simulink model "helicopter"  (R2023b)
settings: Solver=VariableStepAuto  StartTime=0.0  StopTime=20  MaxStep=0.01  RelTol=1e-5
undefined symbols (not defined in the file): A, A_obs, B, B_alt, B_obs, C, C_obs, E_alt, K_act_b, K_act_f, K_f_lqr, K_lqr, L, M_inv_alt, sim_nonlinear, u0, x0
libraries: cstblocks x2, simulink x2
settings Model: Creator=torb  LastModifiedBy=torb

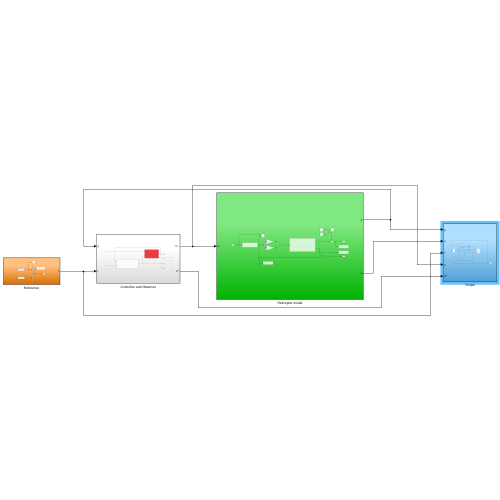
[thumbnail: Simulink's stored preview of the top-level diagram]
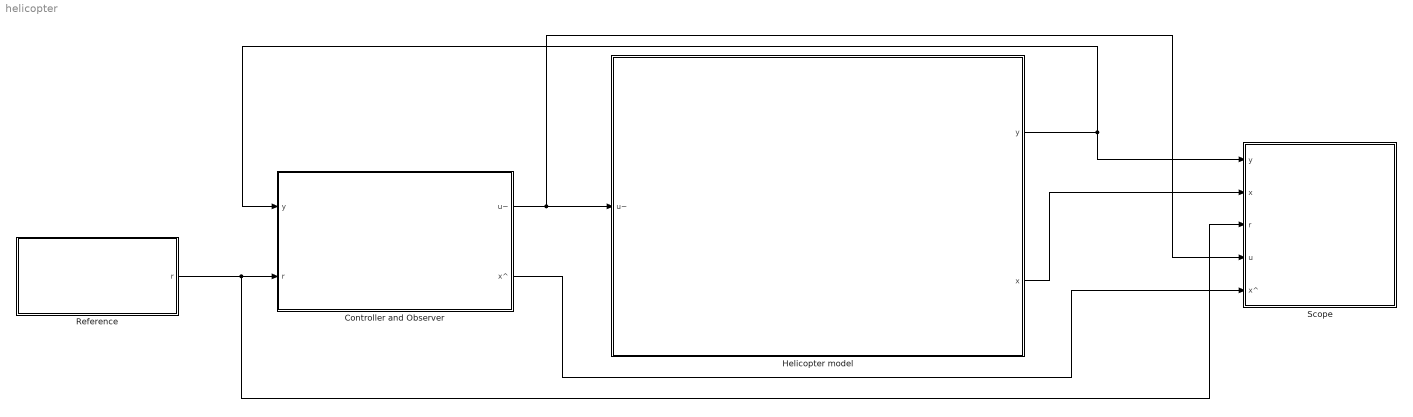
== system helicopter ==
  Controller and Observer : Subsystem
  Helicopter model : Subsystem
  Reference : Subsystem
  Scope : Subsystem
  wires:
  Helicopter model/1(y) -> Scope/1(y), Controller and Observer/1(y)
  Reference/1(r) -> Scope/3(r), Controller and Observer/2(r)
  Helicopter model/2(x) -> Scope/2(x)
  Controller and Observer/1(u~) -> Scope/4(u), Helicopter model/1(u~)
  Controller and Observer/2(x^) -> Scope/5(x^)

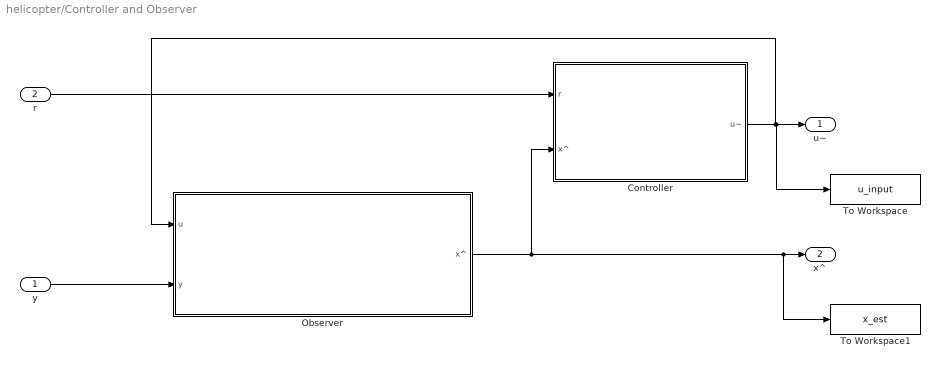
== system helicopter/Controller and Observer ==
  y : Inport
  r : Inport  Port=2
  Controller : Subsystem
  Observer : Subsystem
  To Workspace : ToWorkspace  VariableName=u_input  SaveFormat=Timeseries  SampleTime=-1
  To Workspace1 : ToWorkspace  VariableName=x_est  SaveFormat=Timeseries  SampleTime=-1
  u~ : Outport
  x^ : Outport  Port=2
  wires:
  Controller/1(u~) -> To Workspace/1, u~/1, Observer/1(u)
  Observer/1(x^) -> x^/1, To Workspace1/1, Controller/2(x^)
  r/1 -> Controller/1(r)
  y/1 -> Observer/2(y)

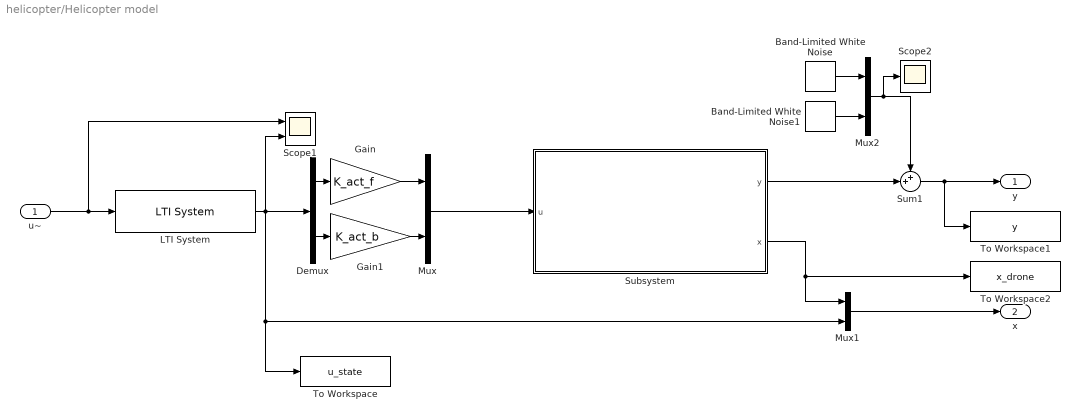
== system helicopter/Helicopter model ==
  u~ : Inport
  Band-Limited White Noise : simulink/Sources/Band-Limited White Noise  Cov=noise_power  Ts=0.01  seed=[23341]
  Band-Limited White Noise1 : simulink/Sources/Band-Limited White Noise  Cov=noise_power  Ts=0.01  seed=[231]
  Demux : Demux  Outputs=2
  Gain : Gain  Gain=K_act_f
  Gain1 : Gain  Gain=K_act_b
  LTI System : cstblocks/LTI System  sys=G_act_real  IC=[]  PadeOrder=0
  Mux : Mux  Inputs=2
  Mux1 : Mux  Inputs=2
  Mux2 : Mux  Inputs=2
  Scope1 : Scope  NumInputPorts=2
  Scope2 : Scope
  Subsystem : Subsystem
  Sum1 : Sum  Inputs=++|
  To Workspace : ToWorkspace  VariableName=u_state  SaveFormat=Timeseries  SampleTime=-1
  To Workspace1 : ToWorkspace  VariableName=y  SaveFormat=Timeseries  SampleTime=-1
  To Workspace2 : ToWorkspace  VariableName=x_drone  SaveFormat=Timeseries  SampleTime=-1
  y : Outport
  x : Outport  Port=2
  wires:
  u~/1 -> LTI System/1, Scope1/1
  LTI System/1 -> Demux/1, Mux1/2, To Workspace/1, Scope1/2
  Demux/2 -> Gain1/1
  Demux/1 -> Gain/1
  Gain/1 -> Mux/1
  Gain1/1 -> Mux/2
  Mux1/1 -> x/1
  Band-Limited White Noise/1 -> Mux2/1
  Band-Limited White Noise1/1 -> Mux2/2
  Mux2/1 -> Sum1/1, Scope2/1
  Sum1/1 -> y/1, To Workspace1/1
  Subsystem/2(x) -> Mux1/1, To Workspace2/1
  Mux/1 -> Subsystem/1(u)
  Subsystem/1(y) -> Sum1/2

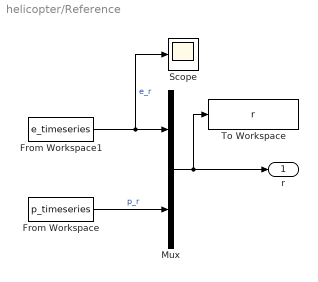
== system helicopter/Reference ==
  From Workspace : FromWorkspace  VariableName=p_timeseries
  From Workspace1 : FromWorkspace  VariableName=e_timeseries
  Mux : Mux  Inputs=2
  Scope : Scope
  To Workspace : ToWorkspace  VariableName=r  SaveFormat=Timeseries  SampleTime=-1
  r : Outport
  wires:
  Mux/1 -> To Workspace/1, r/1
  From Workspace/1 -> Mux/2  "p_r"
  From Workspace1/1 -> Mux/1, Scope/1  "e_r"

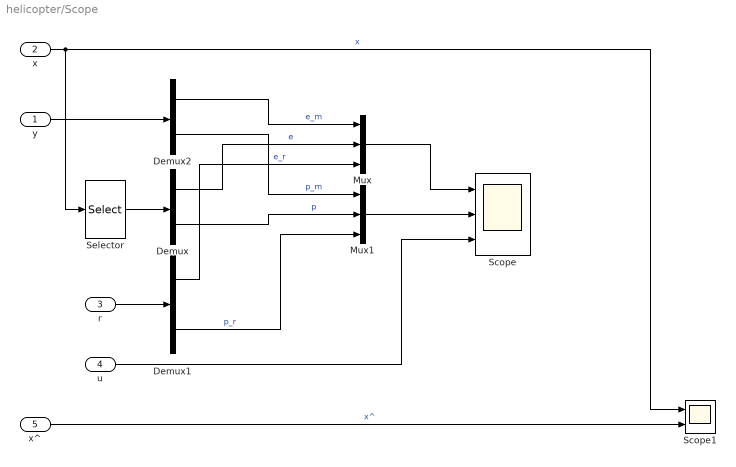
== system helicopter/Scope ==
  y : Inport
  x : Inport  Port=2
  r : Inport  Port=3
  u : Inport  Port=4
  x^ : Inport  Port=5
  Demux : Demux  Outputs=2
  Demux1 : Demux  Outputs=2
  Demux2 : Demux  Outputs=2
  Mux : Mux  Inputs=3
  Mux1 : Mux  Inputs=3
  Scope : Scope  NumInputPorts=3
  Scope1 : Scope  NumInputPorts=2
  Selector : Selector  InputPortWidth=6  IndexOptions=Index vector (dialog)  Indices=[1 2]  OutputSizes=1
  wires:
  r/1 -> Demux1/1
  Mux1/1 -> Scope/2
  Mux/1 -> Scope/1
  x/1 -> Scope1/1, Selector/1  "x"
  x^/1 -> Scope1/2  "x^"
  u/1 -> Scope/3
  Selector/1 -> Demux/1
  y/1 -> Demux2/1
  Demux2/1 -> Mux/1  "e_m"
  Demux2/2 -> Mux1/1  "p_m"
  Demux/1 -> Mux/2  "e"
  Demux/2 -> Mux1/2  "p"
  Demux1/1 -> Mux/3  "e_r"
  Demux1/2 -> Mux1/3  "p_r"

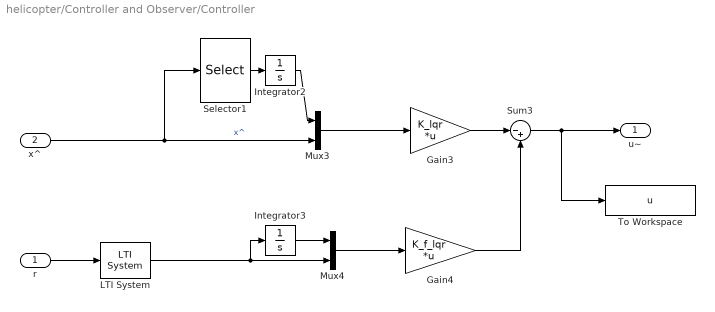
== system helicopter/Controller and Observer/Controller ==
  r : Inport
  x^ : Inport  Port=2
  Gain3 : Gain  Gain=K_lqr  Multiplication=Matrix(K*u)
  Gain4 : Gain  Gain=K_f_lqr  Multiplication=Matrix(K*u)
  Integrator2 : Integrator
  Integrator3 : Integrator
  LTI System : cstblocks/LTI System  sys=ref_filter  IC=[]  PadeOrder=0
  Mux3 : Mux  Inputs=2
  Mux4 : Mux  Inputs=2
  Selector1 : Selector  InputPortWidth=6  IndexOptions=Index vector (dialog)  Indices=[1 2]  OutputSizes=1
  Sum3 : Sum  Inputs=|-+
  To Workspace : ToWorkspace  VariableName=u  SaveFormat=Timeseries  SampleTime=-1
  u~ : Outport
  wires:
  r/1 -> LTI System/1
  LTI System/1 -> Mux4/2, Integrator3/1
  Gain4/1 -> Sum3/2
  Gain3/1 -> Sum3/1
  Sum3/1 -> To Workspace/1, u~/1
  Mux3/1 -> Gain3/1
  Selector1/1 -> Integrator2/1
  Integrator2/1 -> Mux3/1
  x^/1 -> Selector1/1, Mux3/2  "x^"
  Integrator3/1 -> Mux4/1
  Mux4/1 -> Gain4/1

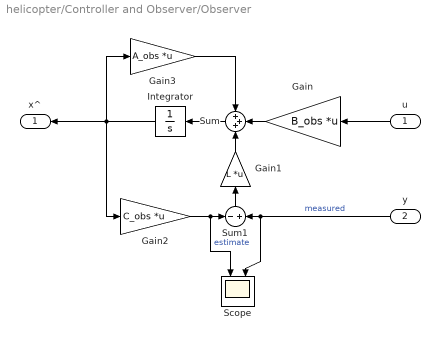
== system helicopter/Controller and Observer/Observer ==
  u : Inport
  y : Inport  Port=2
  Gain : Gain  Gain=B_obs  Multiplication=Matrix(K*u)
  Gain1 : Gain  Gain=L  Multiplication=Matrix(K*u)
  Gain2 : Gain  Gain=C_obs  Multiplication=Matrix(K*u)
  Gain3 : Gain  Gain=A_obs  Multiplication=Matrix(K*u)
  Integrator : Integrator
  Scope : Scope  NumInputPorts=2
  Sum : Sum  Inputs=+++
  Sum1 : Sum  Inputs=-|+
  x^ : Outport
  wires:
  Gain/1 -> Sum/2
  Sum/1 -> Integrator/1
  Integrator/1 -> Gain2/1, x^/1, Gain3/1
  Gain2/1 -> Scope/1, Sum1/1  "estimate"
  Gain1/1 -> Sum/3
  Sum1/1 -> Gain1/1
  Gain3/1 -> Sum/1
  y/1 -> Scope/2, Sum1/2  "measured"
  u/1 -> Gain/1

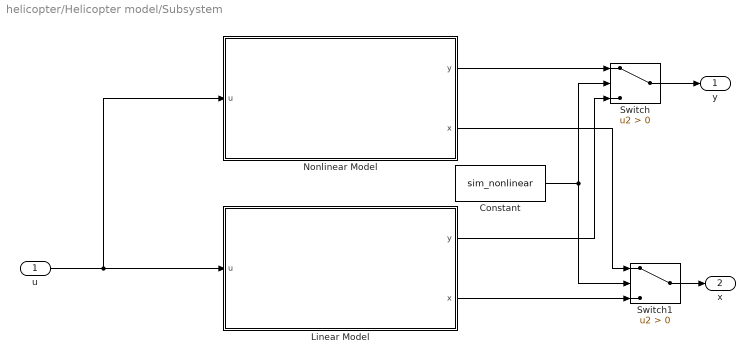
== system helicopter/Helicopter model/Subsystem ==
  u : Inport
  Constant : Constant  Value=sim_nonlinear
  Linear Model : Subsystem
  Nonlinear Model : Subsystem
  Switch : Switch  Criteria=u2 > Threshold  SaturateOnIntegerOverflow=off  InputSameDT=off
  Switch1 : Switch  Criteria=u2 > Threshold  SaturateOnIntegerOverflow=off  InputSameDT=off
  y : Outport
  x : Outport  Port=2
  wires:
  u/1 -> Linear Model/1(u), Nonlinear Model/1(u)
  Switch/1 -> y/1
  Nonlinear Model/1(y) -> Switch/1
  Constant/1 -> Switch1/2, Switch/2
  Switch1/1 -> x/1
  Linear Model/2(x) -> Switch1/3
  Linear Model/1(y) -> Switch/3
  Nonlinear Model/2(x) -> Switch1/1

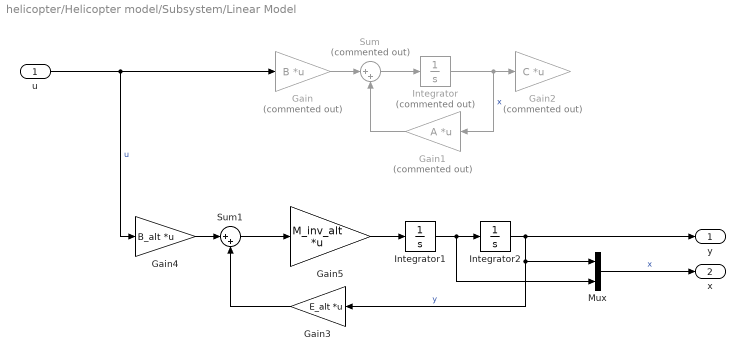
== system helicopter/Helicopter model/Subsystem/Linear Model ==
  u : Inport
  Gain : Gain  Commented=on  Gain=B  Multiplication=Matrix(K*u)
  Gain1 : Gain  Commented=on  Gain=A  Multiplication=Matrix(K*u)
  Gain2 : Gain  Commented=on  Gain=C  Multiplication=Matrix(K*u)
  Gain3 : Gain  Gain=E_alt  Multiplication=Matrix(K*u)
  Gain4 : Gain  Gain=B_alt  Multiplication=Matrix(K*u)
  Gain5 : Gain  Gain=M_inv_alt  Multiplication=Matrix(K*u)
  Integrator : Integrator  Commented=on
  Integrator1 : Integrator
  Integrator2 : Integrator
  Mux : Mux  Inputs=2
  Sum : Sum  Commented=on  Inputs=|++
  Sum1 : Sum  Inputs=|++
  y : Outport
  x : Outport  Port=2
  wires:
  u/1 -> Gain4/1, Gain/1  "u"
  Sum/1 -> Integrator/1
  Gain/1 -> Sum/1
  Gain1/1 -> Sum/2
  Integrator/1 -> Gain1/1, Gain2/1  "x"
  Integrator1/1 -> Integrator2/1, Mux/2
  Integrator2/1 -> y/1, Mux/1, Gain3/1  "y"
  Gain3/1 -> Sum1/2
  Gain4/1 -> Sum1/1
  Sum1/1 -> Gain5/1
  Gain5/1 -> Integrator1/1
  Mux/1 -> x/1  "x"

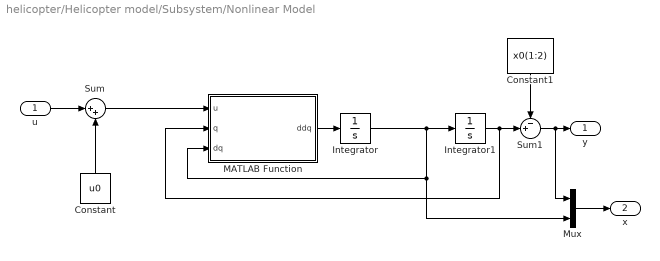
== system helicopter/Helicopter model/Subsystem/Nonlinear Model ==
  u : Inport
  Constant : Constant  Value=u0
  Constant1 : Constant  Value=x0(1:2)
  Integrator : Integrator
  Integrator1 : Integrator  InitialCondition=x0(1:2)
  MATLAB Function : MATLAB Function  TreatAsAtomicUnit=on
  Mux : Mux  Inputs=2
  Sum : Sum  Inputs=|++
  Sum1 : Sum  Inputs=-+|
  y : Outport
  x : Outport  Port=2
  wires:
  Integrator1/1 -> Sum1/2, MATLAB Function/2(q)
  Integrator/1 -> Mux/2, MATLAB Function/3(dq), Integrator1/1
  Mux/1 -> x/1
  MATLAB Function/1(ddq) -> Integrator/1
  u/1 -> Sum/1
  Sum/1 -> MATLAB Function/1(u)
  Constant/1 -> Sum/2
  Constant1/1 -> Sum1/1
  Sum1/1 -> Mux/1, y/1

== matlab function helicopter/Helicopter model/Subsystem/Nonlinear Model/MATLAB Function ==
  data: u input; ddq output size=2; q input; dq input
function ddq = rigid_body_dyn(u, q, dq)
    M = M_fun(q);
    b = b_fun(q, dq);
    g = g_fun(q);
    tau = tau_fun(q, u);

    lam = 0*0.01;
    ddq = (M + lam*eye(size(q, 1)))\(-b-g+tau);
end
